simulink model "FocSpeedGenerator"  (R2024a)
settings: Solver=FixedStepDiscrete  StartTime=0.0  StopTime=10.0  FixedStep=Ts  RelTol=1e-3
values from neighbouring files (symbols this model uses):
  Max_Current = 15    [FocSpeedGeneratorData.mat]
libraries: slpidlib x3
settings Model: Creator=张先生  LastModifiedBy=张先生
settings OptimizationCC: DefaultParameterBehavior=Inlined  UseDivisionForNetSlopeComputation=on  GainParamInheritBuiltInType=on  UseFloatMulNetSlope=on  InlineInvariantSignals=on  PassReuseOutputArgsAs=Individual arguments  ZeroExternalMemoryAtStartup=off  ZeroInternalMemoryAtStartup=off  NoFixptDivByZeroProtection=on  EfficientFloat2IntCast=on  LifeSpan=1  OptimizeBlockOrder=speed  DifferentSizesBufferReuse=on  EfficientTunableParamExpr=on
settings DebuggingCC: ParameterTunabilityLossMsg=error
settings HardwareCC: ProdBitPerPointer=32  ProdBitPerSizeT=32  ProdBitPerPtrDiffT=32  ProdLargestAtomicInteger=Long  ProdLargestAtomicFloat=Double  ProdWordSize=32  ProdLongLongMode=on  ProdHWDeviceType=ARM Compatible->ARM Cortex-M
settings SFSimCC: MATLABDynamicMemAlloc=off
settings RTWCC: Description=Embedded Coder  SystemTargetFile=ert.tlc  TemplateMakefile=ert_default_tmf  GenerateReport=on  LaunchReport=on
settings CodeAppCC: ForceParamTrailComments=on  IgnoreCustomStorageClasses=off  OperatorAnnotations=on  SimulinkDataObjDesc=on  SFDataObjDesc=on  CustomSymbolStrGlobalVar=rt$N$M  CustomSymbolStrType=$N$M  CustomSymbolStrFcn=$N$M$F  CustomSymbolStrMacro=$N$M  InsertBlockDesc=on
settings ERTTargetCC: TargetLangStandard=C99 (ISO)  CodeReplacementLibrary=ARM Cortex-M  GenerateSampleERTMain=on  IncludeMdlTerminateFcn=off  CombineSignalStateStructs=on  SuppressErrorStatus=on  SupportAbsoluteTime=off  SupportComplex=off  InlinedParameterPlacement=NonHierarchical  ERTCustomFileTemplate=example_file_process.tlc  ERTFilePackagingFormat=CompactWithDataFile

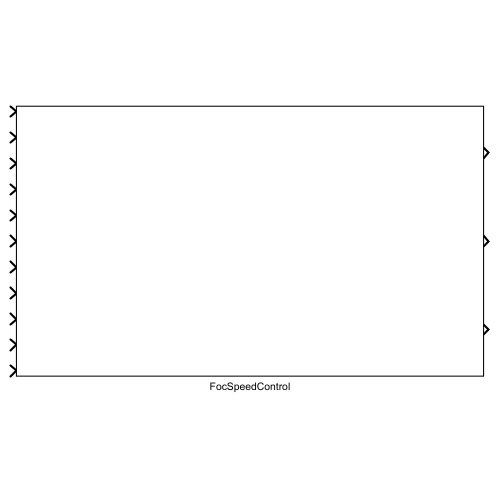
[thumbnail: Simulink's stored preview of the top-level diagram]
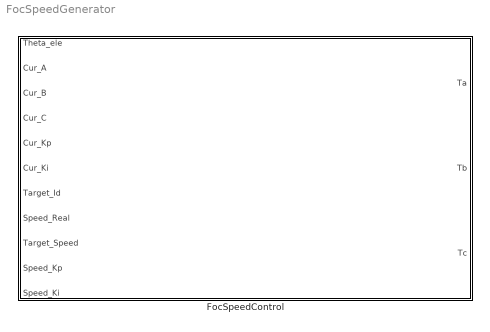
== system FocSpeedGenerator ==
  FocSpeedControl : Subsystem

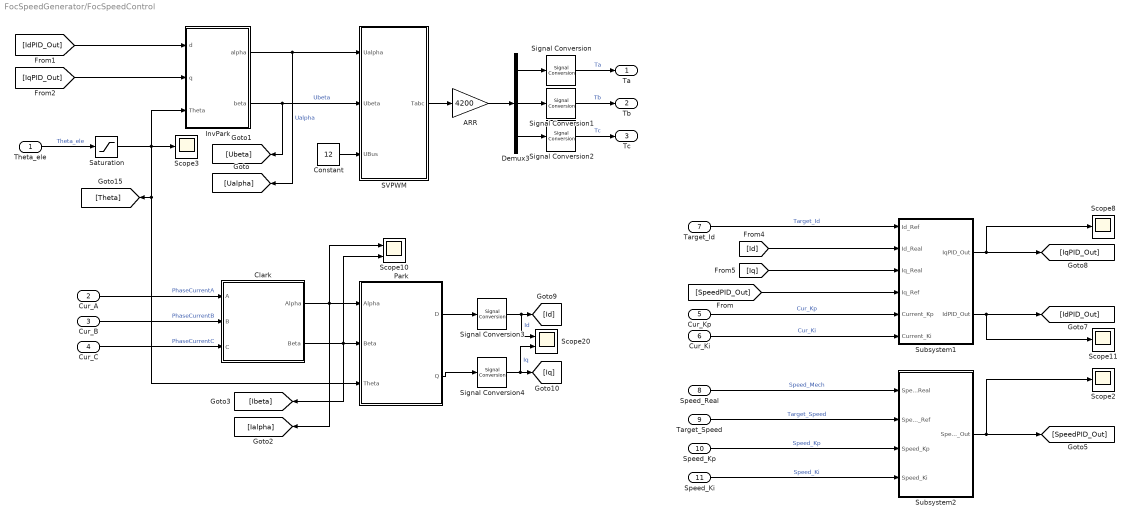
== system FocSpeedGenerator/FocSpeedControl ==
  Theta_ele : Inport
  Cur_A : Inport  Port=2
  Cur_B : Inport  Port=3
  Cur_C : Inport  Port=4
  Cur_Kp : Inport  Port=5
  Cur_Ki : Inport  Port=6
  Target_Id : Inport  Port=7
  Speed_Real : Inport  Port=8
  Target_Speed : Inport  Port=9
  Speed_Kp : Inport  Port=10
  Speed_Ki : Inport  Port=11
  ARR : Gain  Gain=4200
  Clark : Subsystem  TreatAsAtomicUnit=on
      settings: RTWSystemCode=Inline  RTWFcnNameOpts=Use subsystem name
      mask Display:
      | port_label('input',1,'a','texmode','on');
      | port_label('input',2,'b','texmode','on');
      | port_label('input',3,'c','texmode','on');
      | 
      | port_label('output',1,'\alpha','texmode','on');
      | port_label('output',2,'\beta','texmode','on');
      | 
      | fprintf('Clark');
  Constant : Constant  Value=12  OutDataTypeStr=single
  Demux3 : Demux  Outputs=3
  InvPark : Subsystem  TreatAsAtomicUnit=on
      settings: RTWFcnNameOpts=Use subsystem name
      mask Display:
      | port_label('input',1,'d','texmode','on');
      | port_label('input',2,'q','texmode','on');
      | port_label('input',3,'\theta','texmode','on');
      | 
      | port_label('output',1,'\alpha','texmode','on');
      | port_label('output',2,'\beta','texmode','on');
      | 
      | fprintf('Inverse\nPark')
  Park : Subsystem  TreatAsAtomicUnit=on
      settings: RTWFcnNameOpts=Use subsystem name
      mask Display:
      | port_label('input',1,'\alpha','texmode','on');
      | port_label('input',2, '\beta','texmode','on');
      | port_label('input',3, '\theta','texmode','on');
      | 
      | port_label('output',1,'d','texmode','on');
      | port_label('output',2,'q','texmode','on');
      | fprintf('Park');
  SVPWM : Subsystem  TreatAsAtomicUnit=on
  Saturation : Saturate  UpperLimit=2*pi-0.001  LowerLimit=-2*pi + 0.001
  Scope10 : Scope  NumInputPorts=2
  Scope{2..3,8,11} (4 alike) : Scope
  Scope20 : Scope  NumInputPorts=2
  Signal Conversion{,1..4} (5 alike) : SignalConversion  OverrideOpt=off
  Subsystem1 : Subsystem
  Subsystem2 : Subsystem
  Ta : Outport
  Tb : Outport  Port=2
  Tc : Outport  Port=3
  wires:
  [Id] -> Subsystem1/2(Id_Real)
  Clark/2(Beta) -> [Ibeta], Park/2(Beta), Scope10/2
  InvPark/1(alpha) -> SVPWM/1(Ualpha), [Ualpha]  "Ualpha"
  InvPark/2(beta) -> SVPWM/2(Ubeta), [Ubeta]  "Ubeta"
  Saturation/1 -> [Theta], Park/3(Theta), Scope3/1, InvPark/3(Theta)
  Cur_Kp/1 -> Subsystem1/5(Current_Kp)  "Cur_Kp"
  SVPWM/1(Tabc) -> ARR/1
  Subsystem1/1(IqPID_Out) -> Scope8/1, [IqPID_Out]
  Theta_ele/1 -> Saturation/1  "Theta_ele"
  ARR/1 -> Demux3/1
  Cur_C/1 -> Clark/3(C)  "PhaseCurrentC"
  Park/1(D) -> Signal Conversion3/1
  Target_Id/1 -> Subsystem1/1(Id_Ref)  "Target_Id"
  Signal Conversion4/1 -> Scope20/2, [Iq]  "Iq"
  Cur_B/1 -> Clark/2(B)  "PhaseCurrentB"
  [IdPID_Out] -> InvPark/1(d)
  Signal Conversion2/1 -> Tc/1  "Tc"
  Signal Conversion3/1 -> Scope20/1, [Id]  "Id"
  Signal Conversion/1 -> Ta/1  "Ta"
  Cur_A/1 -> Clark/1(A)  "PhaseCurrentA"
  Demux3/2 -> Signal Conversion1/1
  Demux3/1 -> Signal Conversion/1
  Park/2(Q) -> Signal Conversion4/1
  [IqPID_Out] -> InvPark/2(q)
  [Iq] -> Subsystem1/3(Iq_Real)
  Demux3/3 -> Signal Conversion2/1
  Subsystem1/2(IdPID_Out) -> Scope11/1, [IdPID_Out]
  Clark/1(Alpha) -> [Ialpha], Park/1(Alpha), Scope10/1
  Signal Conversion1/1 -> Tb/1  "Tb"
  Constant/1 -> SVPWM/3(UBus)
  Cur_Ki/1 -> Subsystem1/6(Current_Ki)  "Cur_Ki"
  Subsystem2/1(SpeedPID_Out) -> Scope2/1, [SpeedPID_Out]
  [SpeedPID_Out] -> Subsystem1/4(Iq_Ref)
  Speed_Real/1 -> Subsystem2/1(Speed_Real)  "Speed_Mech"
  Target_Speed/1 -> Subsystem2/2(Speed_Ref)  "Target_Speed"
  Speed_Kp/1 -> Subsystem2/3(Speed_Kp)  "Speed_Kp"
  Speed_Ki/1 -> Subsystem2/4(Speed_Ki)  "Speed_Ki"

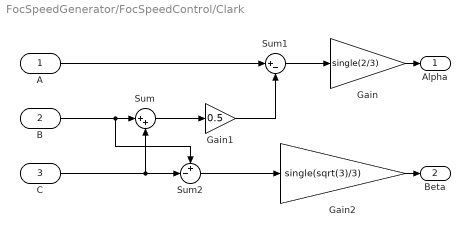
== system FocSpeedGenerator/FocSpeedControl/Clark ==
  A : Inport  OutDataTypeStr=single
  B : Inport  Port=2  OutDataTypeStr=single
  C : Inport  Port=3  OutDataTypeStr=single
  Gain : Gain  Gain=single(2/3)  OutDataTypeStr=single
  Gain1 : Gain  Gain=0.5  OutDataTypeStr=single
  Gain2 : Gain  Gain=single(sqrt(3)/3)  OutDataTypeStr=single
  Sum : Sum  Inputs=|++  OutDataTypeStr=single
  Sum1 : Sum  Inputs=|+-  OutDataTypeStr=single
  Sum2 : Sum  Inputs=+-|  OutDataTypeStr=single
  Alpha : Outport  OutDataTypeStr=single
  Beta : Outport  Port=2  OutDataTypeStr=single
  wires:
  Sum/1 -> Gain1/1
  Gain2/1 -> Beta/1
  B/1 -> Sum2/1, Sum/1
  Gain1/1 -> Sum1/2
  Gain/1 -> Alpha/1
  Sum2/1 -> Gain2/1
  C/1 -> Sum2/2, Sum/2
  A/1 -> Sum1/1
  Sum1/1 -> Gain/1

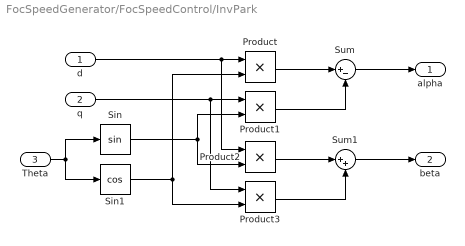
== system FocSpeedGenerator/FocSpeedControl/InvPark ==
  d : Inport  OutDataTypeStr=single
  q : Inport  Port=2  OutDataTypeStr=single
  Theta : Inport  Port=3  OutDataTypeStr=single
  Product{,1..3} (4 alike) : Product  OutDataTypeStr=single
  Sin : Trigonometry  ApproximationMethod=Lookup  TableDataTypeStr=single
  Sin1 : Trigonometry  Operator=cos  ApproximationMethod=Lookup  TableDataTypeStr=single
  Sum : Sum  Inputs=|+-  OutDataTypeStr=single
  Sum1 : Sum  Inputs=|++  OutDataTypeStr=single
  alpha : Outport  OutDataTypeStr=single
  beta : Outport  Port=2  OutDataTypeStr=single
  wires:
  Sum/1 -> alpha/1
  Theta/1 -> Sin1/1, Sin/1
  d/1 -> Product2/1, Product/1
  Sin1/1 -> Product/2, Product3/2
  q/1 -> Product3/1, Product1/1
  Sin/1 -> Product1/2, Product2/2
  Product/1 -> Sum/1
  Product1/1 -> Sum/2
  Product2/1 -> Sum1/1
  Product3/1 -> Sum1/2
  Sum1/1 -> beta/1

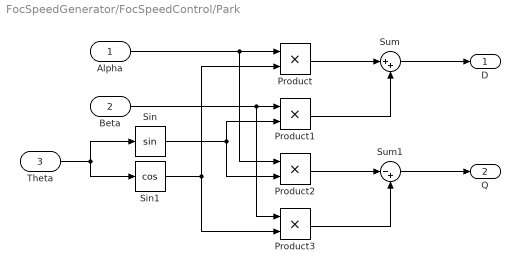
== system FocSpeedGenerator/FocSpeedControl/Park ==
  Alpha : Inport  OutDataTypeStr=single
  Beta : Inport  Port=2  OutDataTypeStr=single
  Theta : Inport  Port=3  OutDataTypeStr=single
  Product{,1..3} (4 alike) : Product  OutDataTypeStr=single
  Sin : Trigonometry  ApproximationMethod=Lookup  TableDataTypeStr=single
  Sin1 : Trigonometry  Operator=cos  ApproximationMethod=Lookup  TableDataTypeStr=single
  Sum : Sum  Inputs=|++  OutDataTypeStr=single
  Sum1 : Sum  Inputs=|-+  OutDataTypeStr=single
  D : Outport  OutDataTypeStr=single
  Q : Outport  Port=2  OutDataTypeStr=single
  wires:
  Beta/1 -> Product3/1, Product1/1
  Alpha/1 -> Product2/1, Product/1
  Theta/1 -> Sin1/1, Sin/1
  Sin1/1 -> Product/2, Product3/2
  Sin/1 -> Product1/2, Product2/2
  Product/1 -> Sum/1
  Product1/1 -> Sum/2
  Sum/1 -> D/1
  Product2/1 -> Sum1/1
  Product3/1 -> Sum1/2
  Sum1/1 -> Q/1

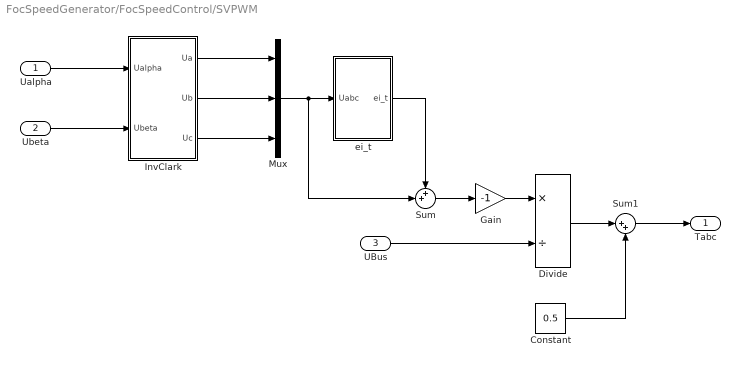
== system FocSpeedGenerator/FocSpeedControl/SVPWM ==
  Ualpha : Inport  OutDataTypeStr=single
  Ubeta : Inport  Port=2  OutDataTypeStr=single
  UBus : Inport  Port=3  OutDataTypeStr=single
  Constant : Constant  Value=0.5  OutDataTypeStr=single
  Divide : Product  Inputs=*/  OutDataTypeStr=single
  Gain : Gain  Gain=-1  OutDataTypeStr=single
  InvClark : Subsystem
  Mux : Mux  Inputs=3
  Sum : Sum  Inputs=++|  OutDataTypeStr=single
  Sum1 : Sum  Inputs=|++  OutDataTypeStr=single
  ei_t : Subsystem
  Tabc : Outport  OutDataTypeStr=single
  wires:
  Ualpha/1 -> InvClark/1(Ualpha)
  Ubeta/1 -> InvClark/2(Ubeta)
  ei_t/1(ei_t) -> Sum/1
  InvClark/1(Ua) -> Mux/1
  InvClark/2(Ub) -> Mux/2
  InvClark/3(Uc) -> Mux/3
  Sum/1 -> Gain/1
  Mux/1 -> Sum/2, ei_t/1(Uabc)
  Divide/1 -> Sum1/1
  Constant/1 -> Sum1/2
  UBus/1 -> Divide/2
  Gain/1 -> Divide/1
  Sum1/1 -> Tabc/1

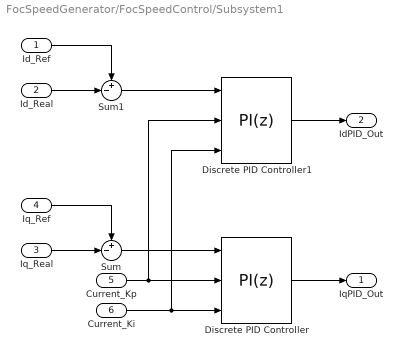
== system FocSpeedGenerator/FocSpeedControl/Subsystem1 ==
  Id_Ref : Inport
  Id_Real : Inport  Port=2
  Iq_Real : Inport  Port=3
  Iq_Ref : Inport  Port=4
  Current_Kp : Inport  Port=5
  Current_Ki : Inport  Port=6
  Discrete PID Controller : slpidlib/PID Controller  Controller=PI  Form=Parallel  TimeDomain=Discrete-time  UseExternalTs=off  SampleTime=-1  IntegratorMethod=Forward Euler  FilterMethod=Forward Euler  ControllerParametersSource=external  P=1  I=1  UseKiTs=off  D=0  UseExternalDerivativeSource=off  N=100  UseFilter=on  TunerSelectOption=Transfer Function Based (PID Tuner App)  InitialConditionSource=internal  InitialConditionForIntegrator=0  InitialConditionForFilter=0  DifferentiatorICPrevScaledInput=0  ExternalReset=none  TrackingMode=off  Kt=1  LimitOutput=on  SatLimitsSource=internal  UpperSaturationLimit=6  LowerSaturationLimit=-6  LinearizeAsGain=off  AntiWindupMode=clamping  Kb=1  LimitIntegrator=off  UpperIntegratorSaturationLimit=inf  LowerIntegratorSaturationLimit=-inf  SaturateOnIntegerOverflow=on  PGainOutDataTypeStr=single  PProdOutDataTypeStr=single  POutMin=[]  POutMax=[]  IGainOutDataTypeStr=single  IProdOutDataTypeStr=single  IOutMin=[]  IOutMax=[]  DOutMin=[]  DOutMax=[]  NOutMin=[]  NOutMax=[]  SumOutDataTypeStr=single  SumOutMin=[]  SumOutMax=[]  SaturationOutMin=[]  SaturationOutMax=[]  PParamMin=[]  PParamMax=[]  IParamMin=[]  IParamMax=[]  DParamMin=[]  DParamMax=[]  NParamMin=[]  NParamMax=[]  KbParamMin=[]  KbParamMax=[]  KtParamMin=[]  KtParamMax=[]  KbOutMin=[]  KbOutMax=[]  KtOutMin=[]  KtOutMax=[]  IntegratorOutMin=[]  IntegratorOutMax=[]  FilterOutMin=[]  FilterOutMax=[]  SumI1OutMin=[]  SumI1OutMax=[]  SumI2OutMin=[]  SumI2OutMax=[]  SumI3OutMin=[]  SumI3OutMax=[]  SumI4OutMin=[]  SumI4OutMax=[]  SumDOutMin=[]  SumDOutMax=[]  DifferentiatorOutMin=[]  DifferentiatorOutMax=[]  FilterDiffOutCoefMin=[]  FilterDiffOutCoefMax=[]  ReciprocalOutMin=[]  ReciprocalOutMax=[]  SumDenOutMin=[]  SumDenOutMax=[]  SumNumOutMin=[]  SumNumOutMax=[]  DivideOutMin=[]  DivideOutMax=[]  UdiffTsProdOutMin=[]  UdiffTsProdOutMax=[]  NTsProdOutMin=[]  NTsProdOutMax=[]  UintegralTsProdOutMin=[]  UintegralTsProdOutMax=[]  UngainTsProdOutMin=[]  UngainTsProdOutMax=[]  ClampingZeroOutDataTypeStr=Inherit: Inherit via back propagation  ClampingZeroOutMin=[]  ClampingZeroOutMax=[]  FilterDenConstantOutDataTypeStr=Inherit: Inherit via back propagation  FilterDenConstantOutMin=[]  FilterDenConstantOutMax=[]  PCopyOutDataTypeStr=Inherit: Inherit via back propagation  PCopyOutMin=[]  PCopyOutMax=[]  NCopyOutDataTypeStr=Inherit: Inherit via back propagation  NCopyOutMin=[]  NCopyOutMax=[]  IntegratorContinuousStateAttributes=''  IntegratorStateMustResolveToSignalObject=off  IntegratorRTWStateStorageClass=Auto  FilterContinuousStateAttributes=''  FilterStateMustResolveToSignalObject=off  FilterRTWStateStorageClass=Auto  ParallelPVariant=ExternalParameters  IdealPVariant=Disabled  IVariant=ExternalParameters  DVariant=Disabled  IntegratorVariant=Discrete  SatVariant=Enabled  AWVariant=DiscClampingParallel  PCopyVariant=Disabled  TRVariant=Disabled  FdbkBlocksVariant=Forward  IdealPFdbkVariant=Disabled  SatFdbkVariant=Disabled  DerivativeFilterVariant=Disabled  NVariant=Disabled  NCopyVariant=Disabled_SignalSpec  FilterICVariant=Disabled  IntegratorICVariant=InternalICs  ExternalResetVariant=Disabled  TRSumVariant=Passthrough  SumFdbkVariant=Disabled  SumVariant=Sum_PI  TsampFilterVariant=InternalTs  TsampNgainVariant=Passthrough  TsampIntegralVariant=Disabled_SignalSpec  ExternalSaturationOutDataTypeStr=Inherit: Same as second input  DerivativeSourceVariant=Disabled
      settings: LibrarySourceBlock=simulink/Discrete/Discrete PID Controller
  Discrete PID Controller1 : slpidlib/PID Controller  Controller=PI  Form=Parallel  TimeDomain=Discrete-time  UseExternalTs=off  SampleTime=-1  IntegratorMethod=Forward Euler  FilterMethod=Forward Euler  ControllerParametersSource=external  P=1  I=1  UseKiTs=off  D=0  UseExternalDerivativeSource=off  N=100  UseFilter=on  TunerSelectOption=Transfer Function Based (PID Tuner App)  InitialConditionSource=internal  InitialConditionForIntegrator=0  InitialConditionForFilter=0  DifferentiatorICPrevScaledInput=0  ExternalReset=none  TrackingMode=off  Kt=1  LimitOutput=on  SatLimitsSource=internal  UpperSaturationLimit=6  LowerSaturationLimit=-6  LinearizeAsGain=off  AntiWindupMode=clamping  Kb=1  LimitIntegrator=off  UpperIntegratorSaturationLimit=inf  LowerIntegratorSaturationLimit=-inf  SaturateOnIntegerOverflow=on  PGainOutDataTypeStr=single  PProdOutDataTypeStr=single  POutMin=[]  POutMax=[]  IGainOutDataTypeStr=single  IProdOutDataTypeStr=single  IOutMin=[]  IOutMax=[]  DOutMin=[]  DOutMax=[]  NOutMin=[]  NOutMax=[]  SumOutDataTypeStr=single  SumOutMin=[]  SumOutMax=[]  SaturationOutMin=[]  SaturationOutMax=[]  PParamMin=[]  PParamMax=[]  IParamMin=[]  IParamMax=[]  DParamMin=[]  DParamMax=[]  NParamMin=[]  NParamMax=[]  KbParamMin=[]  KbParamMax=[]  KtParamMin=[]  KtParamMax=[]  KbOutMin=[]  KbOutMax=[]  KtOutMin=[]  KtOutMax=[]  IntegratorOutMin=[]  IntegratorOutMax=[]  FilterOutMin=[]  FilterOutMax=[]  SumI1OutMin=[]  SumI1OutMax=[]  SumI2OutMin=[]  SumI2OutMax=[]  SumI3OutMin=[]  SumI3OutMax=[]  SumI4OutMin=[]  SumI4OutMax=[]  SumDOutMin=[]  SumDOutMax=[]  DifferentiatorOutMin=[]  DifferentiatorOutMax=[]  FilterDiffOutCoefMin=[]  FilterDiffOutCoefMax=[]  ReciprocalOutMin=[]  ReciprocalOutMax=[]  SumDenOutMin=[]  SumDenOutMax=[]  SumNumOutMin=[]  SumNumOutMax=[]  DivideOutMin=[]  DivideOutMax=[]  UdiffTsProdOutMin=[]  UdiffTsProdOutMax=[]  NTsProdOutMin=[]  NTsProdOutMax=[]  UintegralTsProdOutMin=[]  UintegralTsProdOutMax=[]  UngainTsProdOutMin=[]  UngainTsProdOutMax=[]  ClampingZeroOutDataTypeStr=Inherit: Inherit via back propagation  ClampingZeroOutMin=[]  ClampingZeroOutMax=[]  FilterDenConstantOutDataTypeStr=Inherit: Inherit via back propagation  FilterDenConstantOutMin=[]  FilterDenConstantOutMax=[]  PCopyOutDataTypeStr=Inherit: Inherit via back propagation  PCopyOutMin=[]  PCopyOutMax=[]  NCopyOutDataTypeStr=Inherit: Inherit via back propagation  NCopyOutMin=[]  NCopyOutMax=[]  IntegratorContinuousStateAttributes=''  IntegratorStateMustResolveToSignalObject=off  IntegratorRTWStateStorageClass=Auto  FilterContinuousStateAttributes=''  FilterStateMustResolveToSignalObject=off  FilterRTWStateStorageClass=Auto  ParallelPVariant=ExternalParameters  IdealPVariant=Disabled  IVariant=ExternalParameters  DVariant=Disabled  IntegratorVariant=Discrete  SatVariant=Enabled  AWVariant=DiscClampingParallel  PCopyVariant=Disabled  TRVariant=Disabled  FdbkBlocksVariant=Forward  IdealPFdbkVariant=Disabled  SatFdbkVariant=Disabled  DerivativeFilterVariant=Disabled  NVariant=Disabled  NCopyVariant=Disabled_SignalSpec  FilterICVariant=Disabled  IntegratorICVariant=InternalICs  ExternalResetVariant=Disabled  TRSumVariant=Passthrough  SumFdbkVariant=Disabled  SumVariant=Sum_PI  TsampFilterVariant=InternalTs  TsampNgainVariant=Passthrough  TsampIntegralVariant=Disabled_SignalSpec  ExternalSaturationOutDataTypeStr=Inherit: Same as second input  DerivativeSourceVariant=Disabled
      settings: LibrarySourceBlock=simulink/Discrete/Discrete PID Controller
  Sum : Sum  Inputs=+-|
  Sum1 : Sum  Inputs=+-|
  IqPID_Out : Outport
  IdPID_Out : Outport  Port=2
  wires:
  Sum/1 -> Discrete PID Controller/1
  Current_Kp/1 -> Discrete PID Controller/2, Discrete PID Controller1/2
  Iq_Ref/1 -> Sum/1
  Discrete PID Controller/1 -> IqPID_Out/1
  Current_Ki/1 -> Discrete PID Controller/3, Discrete PID Controller1/3
  Iq_Real/1 -> Sum/2
  Id_Ref/1 -> Sum1/1
  Id_Real/1 -> Sum1/2
  Sum1/1 -> Discrete PID Controller1/1
  Discrete PID Controller1/1 -> IdPID_Out/1

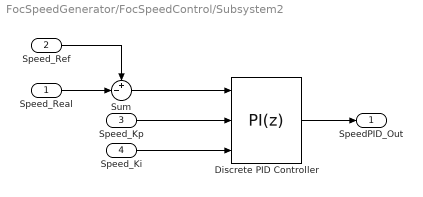
== system FocSpeedGenerator/FocSpeedControl/Subsystem2 ==
  Speed_Real : Inport
  Speed_Ref : Inport  Port=2
  Speed_Kp : Inport  Port=3
  Speed_Ki : Inport  Port=4
  Discrete PID Controller : slpidlib/PID Controller  Controller=PI  Form=Parallel  TimeDomain=Discrete-time  UseExternalTs=off  SampleTime=0.00025  IntegratorMethod=Forward Euler  FilterMethod=Forward Euler  ControllerParametersSource=external  P=1  I=1  UseKiTs=off  D=0  UseExternalDerivativeSource=off  N=100  UseFilter=on  TunerSelectOption=Transfer Function Based (PID Tuner App)  InitialConditionSource=internal  InitialConditionForIntegrator=0  InitialConditionForFilter=0  DifferentiatorICPrevScaledInput=0  ExternalReset=none  TrackingMode=off  Kt=1  LimitOutput=on  SatLimitsSource=internal  UpperSaturationLimit=Max_Current  LowerSaturationLimit=-Max_Current  LinearizeAsGain=off  AntiWindupMode=clamping  Kb=1  LimitIntegrator=off  UpperIntegratorSaturationLimit=inf  LowerIntegratorSaturationLimit=-inf  SaturateOnIntegerOverflow=on  PGainOutDataTypeStr=single  PProdOutDataTypeStr=single  POutMin=[]  POutMax=[]  IGainOutDataTypeStr=single  IProdOutDataTypeStr=single  IOutMin=[]  IOutMax=[]  DOutMin=[]  DOutMax=[]  NOutMin=[]  NOutMax=[]  SumOutDataTypeStr=single  SumOutMin=[]  SumOutMax=[]  SaturationOutMin=[]  SaturationOutMax=[]  PParamMin=[]  PParamMax=[]  IParamMin=[]  IParamMax=[]  DParamMin=[]  DParamMax=[]  NParamMin=[]  NParamMax=[]  KbParamMin=[]  KbParamMax=[]  KtParamMin=[]  KtParamMax=[]  KbOutMin=[]  KbOutMax=[]  KtOutMin=[]  KtOutMax=[]  IntegratorOutMin=[]  IntegratorOutMax=[]  FilterOutMin=[]  FilterOutMax=[]  SumI1OutMin=[]  SumI1OutMax=[]  SumI2OutMin=[]  SumI2OutMax=[]  SumI3OutMin=[]  SumI3OutMax=[]  SumI4OutMin=[]  SumI4OutMax=[]  SumDOutMin=[]  SumDOutMax=[]  DifferentiatorOutMin=[]  DifferentiatorOutMax=[]  FilterDiffOutCoefMin=[]  FilterDiffOutCoefMax=[]  ReciprocalOutMin=[]  ReciprocalOutMax=[]  SumDenOutMin=[]  SumDenOutMax=[]  SumNumOutMin=[]  SumNumOutMax=[]  DivideOutMin=[]  DivideOutMax=[]  UdiffTsProdOutMin=[]  UdiffTsProdOutMax=[]  NTsProdOutMin=[]  NTsProdOutMax=[]  UintegralTsProdOutMin=[]  UintegralTsProdOutMax=[]  UngainTsProdOutMin=[]  UngainTsProdOutMax=[]  ClampingZeroOutDataTypeStr=Inherit: Inherit via back propagation  ClampingZeroOutMin=[]  ClampingZeroOutMax=[]  FilterDenConstantOutDataTypeStr=Inherit: Inherit via back propagation  FilterDenConstantOutMin=[]  FilterDenConstantOutMax=[]  PCopyOutDataTypeStr=Inherit: Inherit via back propagation  PCopyOutMin=[]  PCopyOutMax=[]  NCopyOutDataTypeStr=Inherit: Inherit via back propagation  NCopyOutMin=[]  NCopyOutMax=[]  IntegratorContinuousStateAttributes=''  IntegratorStateMustResolveToSignalObject=off  IntegratorRTWStateStorageClass=Auto  FilterContinuousStateAttributes=''  FilterStateMustResolveToSignalObject=off  FilterRTWStateStorageClass=Auto  ParallelPVariant=ExternalParameters  IdealPVariant=Disabled  IVariant=ExternalParameters  DVariant=Disabled  IntegratorVariant=Discrete  SatVariant=Enabled  AWVariant=DiscClampingParallel  PCopyVariant=Disabled  TRVariant=Disabled  FdbkBlocksVariant=Forward  IdealPFdbkVariant=Disabled  SatFdbkVariant=Disabled  DerivativeFilterVariant=Disabled  NVariant=Disabled  NCopyVariant=Disabled_SignalSpec  FilterICVariant=Disabled  IntegratorICVariant=InternalICs  ExternalResetVariant=Disabled  TRSumVariant=Passthrough  SumFdbkVariant=Disabled  SumVariant=Sum_PI  TsampFilterVariant=InternalTs  TsampNgainVariant=Passthrough  TsampIntegralVariant=Disabled_SignalSpec  ExternalSaturationOutDataTypeStr=Inherit: Same as second input  DerivativeSourceVariant=Disabled
      settings: LibrarySourceBlock=simulink/Discrete/Discrete PID Controller
  Sum : Sum  Inputs=+-|
  SpeedPID_Out : Outport
  wires:
  Sum/1 -> Discrete PID Controller/1
  Speed_Kp/1 -> Discrete PID Controller/2
  Speed_Ref/1 -> Sum/1
  Discrete PID Controller/1 -> SpeedPID_Out/1
  Speed_Ki/1 -> Discrete PID Controller/3
  Speed_Real/1 -> Sum/2

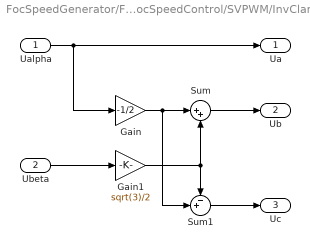
== system FocSpeedGenerator/FocSpeedControl/SVPWM/InvClark ==
  Ualpha : Inport  OutDataTypeStr=single
  Ubeta : Inport  Port=2  OutDataTypeStr=single
  Gain : Gain  Gain=-1/2  OutDataTypeStr=single
  Gain1 : Gain  Gain=sqrt(3)/2  OutDataTypeStr=single
  Sum : Sum  Inputs=|++  OutDataTypeStr=single
  Sum1 : Sum  Inputs=-+|  OutDataTypeStr=single
  Ua : Outport  OutDataTypeStr=single
  Ub : Outport  Port=2  OutDataTypeStr=single
  Uc : Outport  Port=3  OutDataTypeStr=single
  wires:
  Ualpha/1 -> Gain/1, Ua/1
  Ubeta/1 -> Gain1/1
  Gain/1 -> Sum1/2, Sum/1
  Sum/1 -> Ub/1
  Gain1/1 -> Sum/2, Sum1/1
  Sum1/1 -> Uc/1

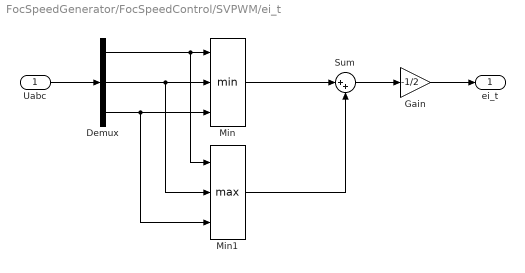
== system FocSpeedGenerator/FocSpeedControl/SVPWM/ei_t ==
  Uabc : Inport  OutDataTypeStr=single
  Demux : Demux  Outputs=3
  Gain : Gain  Gain=-1/2  OutDataTypeStr=single
  Min : MinMax  Inputs=3  OutDataTypeStr=single
  Min1 : MinMax  Function=max  Inputs=3  OutDataTypeStr=single
  Sum : Sum  Inputs=|++  OutDataTypeStr=single
  ei_t : Outport  OutDataTypeStr=single
  wires:
  Min/1 -> Sum/1
  Sum/1 -> Gain/1
  Min1/1 -> Sum/2
  Gain/1 -> ei_t/1
  Uabc/1 -> Demux/1
  Demux/1 -> Min1/1, Min/1
  Demux/2 -> Min/2, Min1/2
  Demux/3 -> Min1/3, Min/3
